simulink model "FM_DEMOD"  (R2021a)
settings: Solver=VariableStepAuto  StartTime=0.0  StopTime=10.0  RelTol=1e-3
libraries: dsparch4 x1, commsynccomp2 x1
settings Model: Creator=Devraj Kashyap  LastModifiedBy=Devraj Kashyap

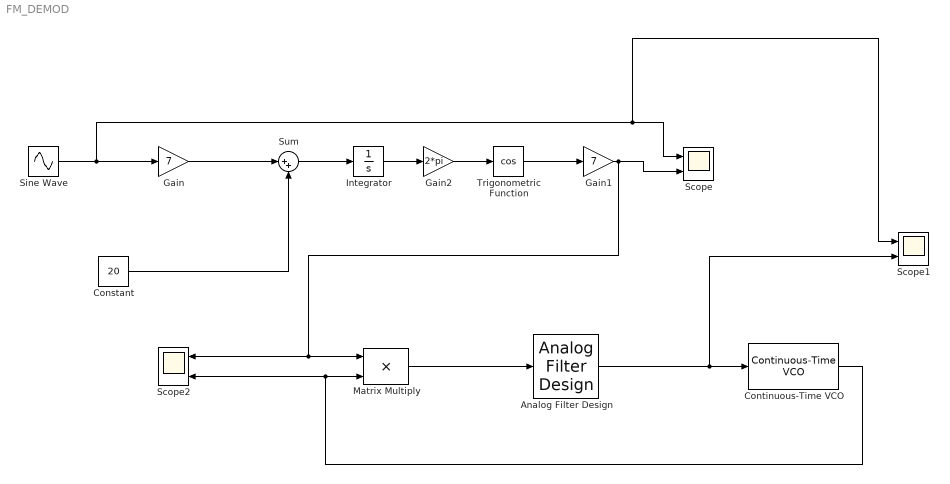
== system FM_DEMOD ==
  Analog Filter Design : dsparch4/Analog Filter Design  method=Butterworth  filttype=Lowpass  N=3  Wlo=2*pi*1  Whi=80  Rp=2  Rs=40
  Constant : Constant  Value=20  SampleTime=0.001
  Continuous-Time VCO : commsynccomp2/Continuous-Time VCO  Ac=1  Fc=100  Kc=10  Ph=0
      settings: SourceProductBaseCode=CM
  Gain : Gain  Gain=7
  Gain1 : Gain  Gain=7
  Gain2 : Gain  Gain=2*pi
  Integrator : Integrator
  Matrix Multiply : Product
  Scope : Scope  NumInputPorts=2
  Scope1 : Scope  NumInputPorts=2
  Scope2 : Scope  NumInputPorts=2
  Sine Wave : Sin  Frequency=2*pi*2  SampleTime=0.001
  Sum : Sum  Inputs=|++
  Trigonometric Function : Trigonometry  Operator=cos
  wires:
  Sine Wave/1 -> Scope1/1, Scope/1, Gain/1
  Constant/1 -> Sum/2
  Gain/1 -> Sum/1
  Sum/1 -> Integrator/1
  Integrator/1 -> Gain2/1
  Gain2/1 -> Trigonometric Function/1
  Trigonometric Function/1 -> Gain1/1
  Gain1/1 -> Scope2/1, Matrix Multiply/1, Scope/2
  Matrix Multiply/1 -> Analog Filter Design/1
  Continuous-Time VCO/1 -> Scope2/2, Matrix Multiply/2
  Analog Filter Design/1 -> Scope1/2, Continuous-Time VCO/1
